simulink model "assignment1_mimo_1"  (R2020b)
settings: Solver=VariableStepAuto  StartTime=0.0  StopTime=500  RelTol=1e-3
values from neighbouring files (symbols this model uses):
  ctr_A = K2.A    [assignment1_mimo1.m]    (also in assignment1_mimo_2.m = K.A)
  ctr_B = K2.B    [assignment1_mimo1.m]    (also in assignment1_mimo_2.m = K.B)
  ctr_C = K2.C    [assignment1_mimo1.m]    (also in assignment1_mimo_2.m = K.C)
  ctr_D = K2.D    [assignment1_mimo1.m]    (also in assignment1_mimo_2.m = K.D)
  GA = Gss.A    [assignment1_mimo1.m]
  GB = Gss.B    [assignment1_mimo1.m]
  GC = Gss.C    [assignment1_mimo1.m]
  GD = Gss.D    [assignment1_mimo1.m]
  GdA = Gdss.A    [assignment1_mimo1.m]
  GdB = Gdss.B    [assignment1_mimo1.m]
  GdC = Gdss.C    [assignment1_mimo1.m]
  GdD = Gdss.D    [assignment1_mimo1.m]
settings Model: Creator=long  LastModifiedBy=long
settings DataIOCC: ReturnWorkspaceOutputs=off

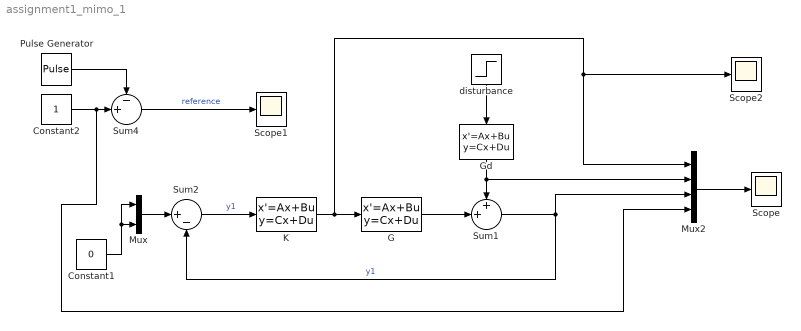
== system assignment1_mimo_1 ==
  Constant1 : Constant  Value=0
  Constant2 : Constant
  G : StateSpace  A=GA  B=GB  C=GC  D=GD  InitialCondition=0
  Gd : StateSpace  A=GdA  B=GdB  C=GdC  D=GdD  InitialCondition=0
  K : StateSpace  A=ctr_A  B=ctr_B  C=ctr_C  D=ctr_D  InitialCondition=0
  Mux : Mux  Inputs=2
  Mux2 : Mux
  Pulse Generator : DiscretePulseGenerator  PulseType=Time based  Amplitude=2  Period=40  PulseWidth=50
  Scope : Scope
  Scope1 : Scope
  Scope2 : Scope
  Sum1 : Sum  Inputs=++|
  Sum2 : Sum  Inputs=|+-
  Sum4 : Sum  Inputs=-+|
  disturbance : Step  Time=15  SampleTime=0
  wires:
  K/1 -> Scope2/1, Mux2/1, G/1
  Constant1/1 -> Mux/1, Mux/2
  Mux2/1 -> Scope/1
  Mux/1 -> Sum2/1
  Sum2/1 -> K/1  "y1"
  Constant2/1 -> Mux2/4, Sum4/2
  Sum4/1 -> Scope1/1  "reference"
  disturbance/1 -> Gd/1
  G/1 -> Sum1/2
  Sum1/1 -> Sum2/2, Mux2/3  "y1"
  Pulse Generator/1 -> Sum4/1
  Gd/1 -> Mux2/2, Sum1/1
